simulink model "intermediate_model"  (R2020a)
settings: Solver=ode45  StartTime=0.0  StopTime=500  MaxStep=40.0  RelTol=1e-9  AbsTol=1e-10
PreLoadFcn:
  | model_startup
model workspace (MAT data in the model file):
  bb_field_prev = Simulink.Parameter
  bb_field_prev.Value = [0; 0; 0]
  bb_field_prev.DataType = 'auto'
  bb_field_prev.Dimensions = [3 1]
  time_prev = Simulink.Parameter
  time_prev.Value = 0
  time_prev.DataType = 'auto'
  time_prev.Dimensions = [1 1]
values from neighbouring files (symbols this model uses):
  b_field = magnetic_field()    [model_startup.m]
  I = (m/12) * diag((y_dim^2 + z_dim^2),(x_dim^2 + z_dim^2),(x_dim^2 + y_dim^2))    [MMOI.m]    (also in euler_eqs.m = MMOI; initialize.m = MMOI; model_startup.m = MMOI)
  X_0 = [q_initial, omega_initial.']    [initialize.m]    (also in model_startup.m = initialize(); test_1.m = [0; 0; 0; init_rates])
settings Model: OrderedModelArguments=off  Creator=Justi  LastModifiedBy=Justi
settings SolverCC: ZeroCrossControl=DisableAll
settings ModelReferenceCC: EnableParallelModelReferenceBuilds=on  ModelReferenceMinAlgLoopOccurrences=on  PropagateSignalLabelsOutOfModel=off
settings RTWCC: BuildConfiguration=Faster Runs

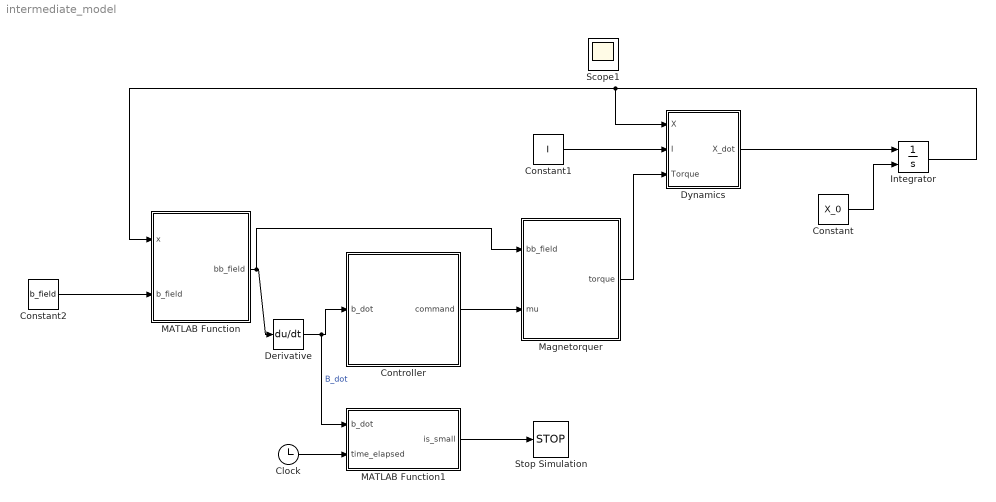
== system intermediate_model ==
  Clock : Clock
  Constant : Constant  Value=X_0  SampleTime=0
  Constant1 : Constant  Value=I
  Constant2 : Constant  Value=b_field
  Controller : MATLAB Function  TreatAsAtomicUnit=on
  Derivative : Derivative
  Dynamics : MATLAB Function  TreatAsAtomicUnit=on
  Integrator : Integrator  InitialConditionSource=external  AbsoluteTolerance=0.000000001  ZeroCross=off
  MATLAB Function : MATLAB Function  TreatAsAtomicUnit=on
  MATLAB Function1 : MATLAB Function  TreatAsAtomicUnit=on
  "Magnetorquer " : MATLAB Function  TreatAsAtomicUnit=on
  Stop Simulation : Stop
  Scope1 : Scope
  wires:
  Dynamics/1(X_dot) -> Integrator/1
  Integrator/1 -> MATLAB Function/1(x), Dynamics/1(X)
  Constant/1 -> Integrator/2
  Constant1/1 -> Dynamics/2(I)
  "Magnetorquer "/1(torque) -> Dynamics/3(Torque)
  Constant2/1 -> MATLAB Function/2(b_field)
  MATLAB Function/1(bb_field) -> "Magnetorquer "/1(bb_field), Derivative/1
  Derivative/1 -> MATLAB Function1/1(b_dot), Controller/1(b_dot)  "B_dot"
  Controller/1(command) -> "Magnetorquer "/2(mu)
  MATLAB Function1/1(is_small) -> Stop Simulation/1
  Clock/1 -> MATLAB Function1/2(time_elapsed)

== matlab function intermediate_model/Dynamics ==
  data: X input; X_dot output; I input; Torque input
function X_dot = EOM(X,I,Torque)
Ix = I(1,1);
Iy = I(2,2);
Iz = I(3,3);
X_dot = EOMS(0,X,Ix,Iy,Iz,Torque);

== matlab function intermediate_model/MATLAB Function ==
  data: x input; bb_field output; b_field input
function bb_field = bb_field_calc(x, b_field)
%bb_field is magnetic field in the body frame
    q = x(1:4);
    C = trans_matrix(quat2eul(q'));
    bb_field = C * b_field;
end

== matlab function intermediate_model/Controller ==
  data: command output; b_dot input
function command = Bang_Bang(b_dot)
    % return the command to the magnetorquer
    command = bang_bang(b_dot);
end

== matlab function intermediate_model/MATLAB Function1 ==
  data: b_dot input; is_small output; time_elapsed input
function is_small = b_dot_mag(b_dot, time_elapsed)

is_small = 0;
tol = 1e-15;

if (norm(b_dot) < tol && time_elapsed > 0)
    is_small = 1;
end

end

== matlab function intermediate_model/Magnetorquer  ==
  data: bb_field input; torque output; mu input
function torque = torque_imparted(bb_field,mu)

%Covering each magnetorquer
%Come back and pull magnetorquer strength from somewhere
m_max = 0.9;
torque = cross(m_max * mu,bb_field);
end
